simulink model "BatteryPowerLimiter"  (R2026b)
settings: Solver=ode45  StopTime=1
settings Model: Creator=Xu Dingyi  LastModifiedBy=29358

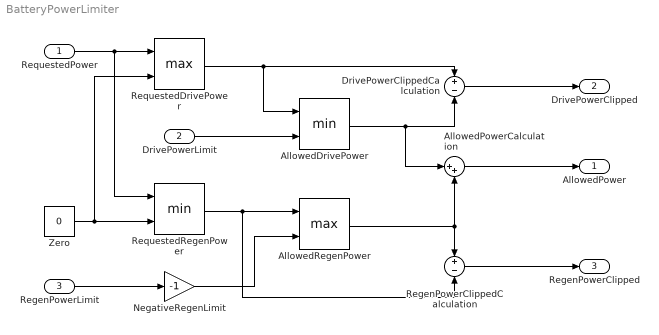
== system BatteryPowerLimiter ==
  RequestedPower : Inport  OutDataTypeStr=double  PortDimensions=1
  DrivePowerLimit : Inport  Port=2  OutDataTypeStr=double  PortDimensions=1
  RegenPowerLimit : Inport  Port=3  OutDataTypeStr=double  PortDimensions=1
  AllowedDrivePower : MinMax  Inputs=2
  AllowedPowerCalculation : Sum  Inputs=|++
  AllowedRegenPower : MinMax  Function=max  Inputs=2
  DrivePowerClippedCalculation : Sum  Inputs=+-
  NegativeRegenLimit : Gain  Gain=-1
  RegenPowerClippedCalculation : Sum  Inputs=+-
  RequestedDrivePower : MinMax  Function=max  Inputs=2
  RequestedRegenPower : MinMax  Inputs=2
  Zero : Constant  Value=0  OutDataTypeStr=double
  AllowedPower : Outport
  DrivePowerClipped : Outport  Port=2
  RegenPowerClipped : Outport  Port=3
  wires:
  RegenPowerClippedCalculation/1 -> RegenPowerClipped/1
  DrivePowerClippedCalculation/1 -> DrivePowerClipped/1
  AllowedPowerCalculation/1 -> AllowedPower/1
  AllowedRegenPower/1 -> AllowedPowerCalculation/2, RegenPowerClippedCalculation/1
  AllowedDrivePower/1 -> AllowedPowerCalculation/1, DrivePowerClippedCalculation/2
  NegativeRegenLimit/1 -> AllowedRegenPower/2
  RequestedRegenPower/1 -> AllowedRegenPower/1, RegenPowerClippedCalculation/2
  RegenPowerLimit/1 -> NegativeRegenLimit/1
  DrivePowerLimit/1 -> AllowedDrivePower/2
  RequestedDrivePower/1 -> AllowedDrivePower/1, DrivePowerClippedCalculation/1
  Zero/1 -> RequestedDrivePower/2, RequestedRegenPower/2
  RequestedPower/1 -> RequestedDrivePower/1, RequestedRegenPower/1
